simulink subsystem "Controls"  (R2024b)
settings: Solver=VariableStepAuto  StartTime=0.0  StopTime=10.0  RelTol=1e-3
undefined symbols (not defined in the file): D1, DiscIntNeverNeededParam, lag, Tctrl, test_alpha, Ts, Yg
libraries: powerlib_extras x74, simulink x10
(part 5 of 7)

== system Controls/fault_trigger/faultgen/faultgen ==
  t : Inport
  Tstat : Inport  Port=2
  Tdur : Inport  Port=3
  Add : Sum
  Logical Operator : Logic  AllPortsSameDT=off  OutDataTypeStr=boolean
  Relational Operator1 : RelationalOperator  Operator=<=  OutDataTypeStr=boolean  InputSameDT=off
  Relational Operatr : RelationalOperator  OutDataTypeStr=boolean  InputSameDT=off
  fault : Outport
  wires:
  Tstat/1 -> Add/1, Relational Operatr/2
  Tdur/1 -> Add/2
  Logical Operator/1 -> fault/1
  t/1 -> Relational Operator1/1, Relational Operatr/1
  Relational Operatr/1 -> Logical Operator/1
  Relational Operator1/1 -> Logical Operator/2
  Add/1 -> Relational Operator1/2

== system Controls/fault_trigger/faultgen/sawtooth ==
  Taqu : Inport
  pules : Inport  Port=2
  Constant : Constant
  Data Type Conversion : DataTypeConversion  SaturateOnIntegerOverflow=off  RndMeth=Floor
  Discrete-Time Integrator : DiscreteIntegrator  ExternalReset=rising  SampleTime=-1  ICPrevOutput=DiscIntNeverNeededParam  ICPrevScaledInput=DiscIntNeverNeededParam
  Logical Operator : Logic  AllPortsSameDT=off
  Relational Operator : RelationalOperator  OutDataTypeStr=boolean  InputSameDT=off
  Unit Delay : UnitDelay  SampleTime=Ts  HasFrameUpgradeWarning=on
  sawtooth : Outport
  trig : Outport  Port=2
  wires:
  Unit Delay/1 -> Relational Operator/1
  Data Type Conversion/1 -> trig/1
  Taqu/1 -> Relational Operator/2
  pules/1 -> Logical Operator/1
  Relational Operator/1 -> Logical Operator/2
  Logical Operator/1 -> Data Type Conversion/1, Discrete-Time Integrator/2
  Discrete-Time Integrator/1 -> sawtooth/1, Unit Delay/1
  Constant/1 -> Discrete-Time Integrator/1

== system Controls/Pole 1 Inverter Control and Protection/Inverter Current //Voltage//Gamma Controller /Current Regulator/Kp Linearisation ==
  note: Kp Linearization
  Alpha_lin : Inport
  Kp : Inport  Port=2
  Inv : Inport  Port=3
  Min_lin : Inport  Port=4
  Max_lin : Inport  Port=5
  Constant3 : Constant  Value=On_lin
  Data Type Conversion : DataTypeConversion  OutDataTypeStr=boolean
  Logical Operator : Logic  Operator=NOT
  Logical Operator1 : Logic  Operator=NOT
  Math Function : Math  Operator=reciprocal  SignedPower=on
  Prod2 : Product  Inputs=3  InputSameDT=on  SaturateOnIntegerOverflow=on  OutDataTypeStr=Inherit: Same as first input
  S6 : Subsystem  mask(Limiter with External Limits){}
      mask Display: disp('      Limiter\n')
  Switch : Switch  Threshold=0.5
  Switch1 : Switch  Threshold=0.5
  Trigonometric Function : Trigonometry
  Trigonometric Function1 : Trigonometry
  k : Gain  Gain=pi/180  SaturateOnIntegerOverflow=on  OutDataTypeStr=Inherit: Same as input  ParamDataTypeStr=Inherit: Same as input
  k1 : Gain  Gain=pi/180  SaturateOnIntegerOverflow=on  OutDataTypeStr=Inherit: Same as input  ParamDataTypeStr=Inherit: Same as input
  Kp_lin : Outport  InitialOutput=0
  wires:
  Data Type Conversion/1 -> Logical Operator1/1
  Constant3/1 -> Data Type Conversion/1
  Min_lin/1 -> S6/3(MIN), Switch/1
  Max_lin/1 -> S6/1(MAX), Switch/3
  Alpha_lin/1 -> S6/2(In)
  Math Function/1 -> Prod2/2
  Trigonometric Function1/1 -> Math Function/1
  k/1 -> Trigonometric Function1/1
  Kp/1 -> Prod2/3, Switch1/1
  Inv/1 -> Logical Operator/1
  Logical Operator/1 -> Switch/2
  Trigonometric Function/1 -> Prod2/1
  S6/1("  ") -> k/1
  k1/1 -> Trigonometric Function/1
  Switch/1 -> k1/1
  Switch1/1 -> Kp_lin/1
  Prod2/1 -> Switch1/3
  Logical Operator1/1 -> Switch1/2  "Off"

== system Controls/Pole 1 Inverter Control and Protection/Inverter Current //Voltage//Gamma Controller /Current Regulator/S16 ==
  note: INTEGRATOR with External limits & Reset & Hold
  note: Gain * dt
  Max : Inport
  Min : Inport  Port=2
  In : Inport  Port=3
  Reset : Inport  Port=4
  Hold : Inport  Port=5
  Reset Value : Inport  Port=6
  Gain1 : Gain  Gain=k*dt  SaturateOnIntegerOverflow=on  OutDataTypeStr=Inherit: Same as input  ParamDataTypeStr=Inherit: Same as input
  IC = ic : UnitDelay  InitialCondition=ic  SampleTime=dt  HasFrameUpgradeWarning=on
  Logical Operator4 : Logic  Operator=OR
  MinMax : MinMax  Inputs=2  InputSameDT=on  SaturateOnIntegerOverflow=on
  MinMax1 : MinMax  Function=max  Inputs=2  InputSameDT=on  SaturateOnIntegerOverflow=on
  S6 : Subsystem  mask(Limiter with External Limits){}
      mask Display: disp('      Limiter\n')
  Sum : Sum  InputSameDT=on  SaturateOnIntegerOverflow=on  OutDataTypeStr=Inherit: Same as first input
  Switch2 : Switch  Threshold=0.5
  Switch3 : Switch  Threshold=0.5
  Switch7 : Switch  Threshold=0.5
  Out : Outport  InitialOutput=0
  wires:
  Gain1/1 -> Sum/1
  In/1 -> Gain1/1
  Sum/1 -> S6/2(In)
  S6/1("  ") -> Out/1, IC = ic/1
  Hold/1 -> Logical Operator4/1
  Reset/1 -> Switch7/2, Logical Operator4/2
  Logical Operator4/1 -> Switch2/2, Switch3/2
  Switch2/1 -> MinMax/1
  Max/1 -> Switch2/3, MinMax/2
  Reset Value/1 -> Switch7/1
  MinMax/1 -> S6/1(MAX)
  MinMax1/1 -> S6/3(MIN)
  Switch3/1 -> MinMax1/1
  Min/1 -> Switch3/3, MinMax1/2
  IC = ic/1 -> Switch7/3
  Switch7/1 -> Switch2/1, Sum/2, Switch3/1

== system Controls/Pole 1 Inverter Control and Protection/Inverter Current //Voltage//Gamma Controller /Current Regulator/S6 ==
  note: Limiter
      | with external
      | limits
  MAX : Inport
  In : Inport  Port=2
  MIN : Inport  Port=3
  MinMax : MinMax  Function=max  Inputs=2  InputSameDT=on  SaturateOnIntegerOverflow=on
  MinMax1 : MinMax  Inputs=2  InputSameDT=on  SaturateOnIntegerOverflow=on
  "  " : Outport  InitialOutput=0
  wires:
  In/1 -> MinMax1/2
  MinMax/1 -> "  "/1
  MIN/1 -> MinMax/1
  MAX/1 -> MinMax1/1
  MinMax1/1 -> MinMax/2

== system Controls/Pole 1 Inverter Control and Protection/Inverter Current //Voltage//Gamma Controller /Gamma Error/S6 ==
  note: Limiter
      | with external
      | limits
  MAX : Inport
  In : Inport  Port=2
  MIN : Inport  Port=3
  MinMax : MinMax  Function=max  Inputs=2  InputSameDT=on  SaturateOnIntegerOverflow=on
  MinMax1 : MinMax  Inputs=2  InputSameDT=on  SaturateOnIntegerOverflow=on
  "  " : Outport  InitialOutput=0
  wires:
  MinMax1/1 -> MinMax/2
  MAX/1 -> MinMax1/1
  MIN/1 -> MinMax/1
  MinMax/1 -> "  "/1
  In/1 -> MinMax1/2

== system Controls/Pole 1 Inverter Control and Protection/Inverter Current //Voltage//Gamma Controller /Gamma Regulator/Gamma Regulator ==
  note: PI Regulator With external limits (Linearized Kp) (Discrete)
  Max_i : Inport
  Min_i : Inport  Port=2
  ERR : Inport  Port=3
  Max_pi : Inport  Port=4
  Min_pi : Inport  Port=5
  Alpha_lin : Inport  Port=6
  Max_lin : Inport  Port=7
  Min_lin : Inport  Port=8
  Inv : Inport  Port=9
  Kp : Inport  Port=10
  Ki : Inport  Port=11
  Ground : Ground
  KI (deg per pu per s) : Gain  Gain=Ki  SaturateOnIntegerOverflow=on  OutDataTypeStr=Inherit: Same as input  ParamDataTypeStr=Inherit: Same as input
  Kp (deg per pu) : Constant  Value=Kp
  Kp Linearisation : Subsystem
  Prod : Product  InputSameDT=on  SaturateOnIntegerOverflow=on  OutDataTypeStr=Inherit: Same as first input
  Prod1 : Product  InputSameDT=on  SaturateOnIntegerOverflow=on  OutDataTypeStr=Inherit: Same as first input
  S16 : Subsystem  mask(Integrator  With  External  Dynamic  Limits (Discrete)){k=1, ic=IC_i, st=pas}
      mask prompts: k "Gain:"; ic "Initial Condition:"; st "Sample time: (s)"
      mask Display: disp('Integrator\nwith\nExternal Limits\nGain & Reset & Hold\n(Discrete)')
  S6 : Subsystem  mask(Limiter with External Limits){}
      mask Display: disp('      Limiter\n')
  Sum : Sum  InputSameDT=on  SaturateOnIntegerOverflow=on  OutDataTypeStr=Inherit: Same as first input
  Alpha_ord : Outport  InitialOutput=0
  wires:
  Prod1/1 -> S16/3(In)
  Ki/1 -> Prod1/2
  Kp/1 -> Kp Linearisation/2(Kp)
  Alpha_lin/1 -> Kp Linearisation/1(Alpha_lin)
  S6/1("  ") -> Alpha_ord/1
  Kp Linearisation/1(Kp_lin) -> Prod/1
  Max_i/1 -> S16/1(Max)
  Min_i/1 -> S16/2(Min)
  Sum/1 -> S6/2(In)
  Max_pi/1 -> S6/1(MAX)
  Min_pi/1 -> S6/3(MIN)
  S16/1(Out) -> Sum/2
  ERR/1 -> Prod1/1, KI (deg per pu per s)/1, Prod/2
  Ground/1 -> S16/4(Reset), S16/5(Hold), S16/6(Reset Value)
  Inv/1 -> Kp Linearisation/3(Inv)
  Max_lin/1 -> Kp Linearisation/5(Max_lin)
  Min_lin/1 -> Kp Linearisation/4(Min_lin)
  Prod/1 -> Sum/1

== system Controls/Pole 1 Inverter Control and Protection/Inverter Current //Voltage//Gamma Controller /Voltage Dependant Current Order Limiter/PB_R ==
  note: Silvano Casoria
      | Laboratoire simulation de reseaux, IREQ
  note: LOW PASS Filter & RESET
      | (Zoh methode)
  "In " : Inport
  Reset : Inport  Port=2
  T : Inport  Port=3
  Constant : Constant  Value=dt
  IC= ic : UnitDelay  InitialCondition=ic  SampleTime=dt  HasFrameUpgradeWarning=on
  Math Function : Math  Operator=reciprocal  SignedPower=on
  Product : Product  Inputs=3  InputSameDT=on  SaturateOnIntegerOverflow=on  OutDataTypeStr=Inherit: Same as first input
  Sum : Sum  Inputs=+-  InputSameDT=on  SaturateOnIntegerOverflow=on  OutDataTypeStr=Inherit: Same as first input
  Sum1 : Sum  InputSameDT=on  SaturateOnIntegerOverflow=on
  Switch : Switch  Threshold=0.5
  Out : Outport  InitialOutput=0
  wires:
  IC= ic/1 -> Sum/2, Sum1/2
  "In "/1 -> Sum/1, Switch/1
  Reset/1 -> Switch/2
  Sum1/1 -> Out/1, Switch/3
  Switch/1 -> IC= ic/1
  Product/1 -> Sum1/1
  Sum/1 -> Product/2
  Math Function/1 -> Product/1
  T/1 -> Math Function/1
  Constant/1 -> Product/3

== system Controls/Pole 1 Inverter Control and Protection/Inverter Current //Voltage//Gamma Controller /Voltage Error/S6 ==
  note: Limiter
      | with external
      | limits
  MAX : Inport
  In : Inport  Port=2
  MIN : Inport  Port=3
  MinMax : MinMax  Function=max  Inputs=2  InputSameDT=on  SaturateOnIntegerOverflow=on
  MinMax1 : MinMax  Inputs=2  InputSameDT=on  SaturateOnIntegerOverflow=on
  "  " : Outport  InitialOutput=0
  wires:
  In/1 -> MinMax1/2
  MinMax/1 -> "  "/1
  MIN/1 -> MinMax/1
  MAX/1 -> MinMax1/1
  MinMax1/1 -> MinMax/2

== system Controls/Pole 1 Inverter Control and Protection/Inverter Current //Voltage//Gamma Controller /Voltage Regulator/Voltage Regulator ==
  note: PI Regulator With external limits (Linearized Kp) (Discrete)
  Max_i : Inport
  Min_i : Inport  Port=2
  ERR : Inport  Port=3
  Max_pi : Inport  Port=4
  Min_pi : Inport  Port=5
  Alpha_lin : Inport  Port=6
  Max_lin : Inport  Port=7
  Min_lin : Inport  Port=8
  Inv : Inport  Port=9
  Kp : Inport  Port=10
  Ki : Inport  Port=11
  Ground : Ground
  KI (deg per pu per s) : Gain  Gain=Ki  SaturateOnIntegerOverflow=on  OutDataTypeStr=Inherit: Same as input  ParamDataTypeStr=Inherit: Same as input
  Kp (deg per pu) : Constant  Value=Kp
  Kp Linearisation : Subsystem
  Prod : Product  InputSameDT=on  SaturateOnIntegerOverflow=on  OutDataTypeStr=Inherit: Same as first input
  Prod1 : Product  InputSameDT=on  SaturateOnIntegerOverflow=on  OutDataTypeStr=Inherit: Same as first input
  S16 : Subsystem  mask(Integrator  With  External  Dynamic  Limits (Discrete)){k=1, ic=IC_i, st=pas}
      mask prompts: k "Gain:"; ic "Initial Condition:"; st "Sample time: (s)"
      mask Display: disp('Integrator\nwith\nExternal Limits\nGain & Reset & Hold\n(Discrete)')
  S6 : Subsystem  mask(Limiter with External Limits){}
      mask Display: disp('      Limiter\n')
  Sum : Sum  InputSameDT=on  SaturateOnIntegerOverflow=on  OutDataTypeStr=Inherit: Same as first input
  Alpha_ord : Outport  InitialOutput=0
  wires:
  Prod1/1 -> S16/3(In)
  Ki/1 -> Prod1/2
  Kp/1 -> Kp Linearisation/2(Kp)
  Prod/1 -> Sum/1
  Min_lin/1 -> Kp Linearisation/4(Min_lin)
  Max_lin/1 -> Kp Linearisation/5(Max_lin)
  Inv/1 -> Kp Linearisation/3(Inv)
  Ground/1 -> S16/6(Reset Value), S16/5(Hold), S16/4(Reset)
  ERR/1 -> Prod1/1, Prod/2, KI (deg per pu per s)/1
  S16/1(Out) -> Sum/2
  Min_pi/1 -> S6/3(MIN)
  Max_pi/1 -> S6/1(MAX)
  Sum/1 -> S6/2(In)
  Min_i/1 -> S16/2(Min)
  Max_i/1 -> S16/1(Max)
  Kp Linearisation/1(Kp_lin) -> Prod/1
  S6/1("  ") -> Alpha_ord/1
  Alpha_lin/1 -> Kp Linearisation/1(Alpha_lin)

== system Controls/Pole 1 Inverter Control and Protection/Inverter Protections/Commutation Failure Prevention Control (CFPREV)/Enabled Subsystem ==
  note: Fast initialisation
      | for simulation
  note: Commutation failure Prevention Control (CFPREV)
  note: Silvano Casoria
      | Power System Laboratory, IREQ
      | Hydro-Quebec
  note: Ref. "A Novel Method to Mitigate Commutation Failures in HVDC Systems,"
      | Lidong Zhang, Lars Dofnas ABB Utilities Power System Technology,
      | Proceedings PowerCon 2002, Volume: 1 , 13-17 Oct. 2002,  Page(s): 51-56 vol.1
  Uabc (pu) : Inport
  Enable : EnablePort
  AB_LEVEL : Constant  Value=ab_level
  ALPFA_BETA_SUM : Fcn  Expr=sqrt(u[1]^2+u[2]^2)
  ALPFA_BETA_SUM1 : Fcn  Expr=abs(u[3]) * 3
  C : Constant  Value=filt_tc
  C1 : Constant  Value=1/(fn)
  CLARK : Subsystem
  Gain : Gain  Gain=ab_gain  SaturateOnIntegerOverflow=on  OutDataTypeStr=Inherit: Same as input  ParamDataTypeStr=Inherit: Same as input
  "Gain  " : Gain  Gain=z_gain  SaturateOnIntegerOverflow=on  OutDataTypeStr=Inherit: Same as input  ParamDataTypeStr=Inherit: Same as input
  Ground : Ground
  LP T= 0.03 : powerlib_extras/Discrete  Control Blocks/Discrete 1st-Order Filter  FilterType=Lowpass  Tc=0.03  Ts=Ts  Initialize=off  Vac_Init=[0.8 -25 60]*0  Vdc_Init=filt_ic  PlotResponse=off  param1=[1 500 0.1]
  Max: 1 pu Min = 0 : Saturate  UpperLimit=1.0  LowerLimit=0
  MinMax2 : MinMax  Function=max  InputSameDT=on  SaturateOnIntegerOverflow=on
  MinMax3 : MinMax  Function=max  Inputs=2  InputSameDT=on  SaturateOnIntegerOverflow=on
  MinMax4 : MinMax  Function=max  Inputs=2  InputSameDT=on  SaturateOnIntegerOverflow=on
  MinMax5 : MinMax  Function=max  InputSameDT=on  SaturateOnIntegerOverflow=on
  PB_R : Subsystem  mask(Low Pass Filter With Reset (discrete: Zoh method, Forward Euler)){ic=1, dt=Ts}
      mask prompts: ic "Initial condition:"; dt "Sample time (s)"
      mask help:
      | The output will be reset to the input value (Time constant = 0)  during the input (2) is True. The Time constant (T) is defined by
      | input (3).
      mask Display:
      | plot(0,0,100,100,[90,80,70,60,50,40,29,20,10],[60,55,52,55,60,65,67,65,60],[89,80,71,60,50,40,30,20,10],[40,35,32,35,40,45,47,45,40],[56,44],[70,50]);
      | disp('\n\nD')
  Relational Operator : RelationalOperator  Operator=>  InputSameDT=off
  Relational Operator1 : RelationalOperator  Operator=>  InputSameDT=off
  Sum : Sum  Inputs=+-  SaturateOnIntegerOverflow=on
  Switch : Switch  Threshold=0.5  InputSameDT=off
  Switch1 : Switch  Threshold=0.5  InputSameDT=off
  Switch2 : Switch  Threshold=0.5  InputSameDT=off
  T_ss : Step  Time=T_ss  Before=1  After=0  SampleTime=Ts
  Tapped Delay : simulink/Discrete/Tapped Delay  vinit=0.0  samptime=Ts  NumDelays=fix(T_periode/Ts)  DelayOrder=Newest  includeCurrent=off
  Tapped Delay1 : simulink/Discrete/Tapped Delay  vinit=0.0  samptime=Ts  NumDelays=fix(T_periode/Ts)  DelayOrder=Newest  includeCurrent=off
  ZERO : Constant  Value=0
  ZERO1 : Constant  Value=0
  Z_LEVEL : Constant  Value=z_level
  AMIN_CFPREV (deg) : Outport
  wires:
  Tapped Delay/1 -> MinMax5/1
  Ground/1 -> PB_R/2(Reset)
  C1/1 -> Switch2/1
  T_ss/1 -> Switch2/2
  C/1 -> Switch2/3
  Switch2/1 -> PB_R/3(T)
  PB_R/1(Out) -> Sum/1
  Uabc (pu)/1 -> CLARK/1(abc)
  CLARK/1(ab0) -> ALPFA_BETA_SUM1/1, ALPFA_BETA_SUM/1
  Switch1/1 -> MinMax3/2  "Z MIN"
  Switch/1 -> MinMax3/1  "AB MIN"
  ZERO1/1 -> Switch1/3
  "Gain  "/1 -> Switch1/1  "Z_AMIN"
  Relational Operator1/1 -> Switch1/2  "Z_DET"
  Max: 1 pu Min = 0/1 -> "Gain  "/1
  MinMax2/1 -> Max: 1 pu Min = 0/1
  Tapped Delay1/1 -> MinMax2/1
  Z_LEVEL/1 -> Relational Operator1/2
  ALPFA_BETA_SUM1/1 -> Tapped Delay1/1, Relational Operator1/1  "Z_DIFF"
  ZERO/1 -> Switch/3
  Gain/1 -> Switch/1  "AB_AMIN"
  MinMax5/1 -> Gain/1
  Relational Operator/1 -> Switch/2  "AB_DET"
  AB_LEVEL/1 -> Relational Operator/2
  Sum/1 -> Tapped Delay/1, Relational Operator/1
  ALPFA_BETA_SUM/1 -> PB_R/1("In "), Sum/2
  MinMax3/1 -> MinMax4/2, LP T= 0.03/1
  LP T= 0.03/1 -> MinMax4/1
  MinMax4/1 -> AMIN_CFPREV (deg)/1

== system Controls/Pole 1 Inverter Control and Protection/Inverter Protections/Low AC Voltage Detection (LACVD)/Enabled Subsystem ==
  note: Low AC Voltage Detection
  note: Silvano Casoria
      | Power System Laboratory, IREQ
      | Hydro-Quebec
  Uac (pu) : Inport
  "Off Delay " : powerlib_extras/Discrete  Control Blocks/Discrete On//Off Delay  type_delay=Off delay  delay=0.009  ic=0  Ts=dt
  On Delay : powerlib_extras/Discrete  Control Blocks/Discrete On//Off Delay  type_delay=On delay  delay=0.014  ic=0  Ts=dt
  "On Delay " : powerlib_extras/Discrete  Control Blocks/Discrete On//Off Delay  type_delay=On delay  delay=0.001  ic=0  Ts=dt
  REF 1 (pu) : Constant  Value=Ref_1
  Relational Operator1 : RelationalOperator  Operator=<=
  Low_AC_Voltage : Outport
  wires:
  Uac (pu)/1 -> Relational Operator1/1
  On Delay/1 -> Low_AC_Voltage/1
  REF 1 (pu)/1 -> Relational Operator1/2
  "Off Delay "/1 -> On Delay/1
  "On Delay "/1 -> "Off Delay "/1
  Relational Operator1/1 -> "On Delay "/1

== system Controls/Pole 1 Rectifier Control and Protection/Rectifier Controller/Current Regulator/Kp Linearisation ==
  note: Kp Linearization
  Alpha_lin : Inport
  Kp : Inport  Port=2
  Inv : Inport  Port=3
  Min_lin : Inport  Port=4
  Max_lin : Inport  Port=5
  Constant3 : Constant  Value=On_lin
  Data Type Conversion : DataTypeConversion  OutDataTypeStr=boolean
  Logical Operator : Logic  Operator=NOT
  Logical Operator1 : Logic  Operator=NOT
  Math Function : Math  Operator=reciprocal  SignedPower=on
  Prod2 : Product  Inputs=3  InputSameDT=on  SaturateOnIntegerOverflow=on  OutDataTypeStr=Inherit: Same as first input
  S6 : Subsystem  mask(Limiter with External Limits){}
      mask Display: disp('      Limiter\n')
  Switch : Switch  Threshold=0.5
  Switch1 : Switch  Threshold=0.5
  Trigonometric Function : Trigonometry
  Trigonometric Function1 : Trigonometry
  k : Gain  Gain=pi/180  SaturateOnIntegerOverflow=on  OutDataTypeStr=Inherit: Same as input  ParamDataTypeStr=Inherit: Same as input
  k1 : Gain  Gain=pi/180  SaturateOnIntegerOverflow=on  OutDataTypeStr=Inherit: Same as input  ParamDataTypeStr=Inherit: Same as input
  Kp_lin : Outport  InitialOutput=0
  wires:
  Data Type Conversion/1 -> Logical Operator1/1
  Constant3/1 -> Data Type Conversion/1
  Min_lin/1 -> S6/3(MIN), Switch/1
  Max_lin/1 -> S6/1(MAX), Switch/3
  Alpha_lin/1 -> S6/2(In)
  Math Function/1 -> Prod2/2
  Trigonometric Function1/1 -> Math Function/1
  k/1 -> Trigonometric Function1/1
  Kp/1 -> Prod2/3, Switch1/1
  Inv/1 -> Logical Operator/1
  Logical Operator/1 -> Switch/2
  Trigonometric Function/1 -> Prod2/1
  S6/1("  ") -> k/1
  k1/1 -> Trigonometric Function/1
  Switch/1 -> k1/1
  Switch1/1 -> Kp_lin/1
  Prod2/1 -> Switch1/3
  Logical Operator1/1 -> Switch1/2  "Off"

== system Controls/Pole 1 Rectifier Control and Protection/Rectifier Controller/Current Regulator/S16 ==
  note: INTEGRATOR with External limits & Reset & Hold
  note: Gain * dt
  Max : Inport
  Min : Inport  Port=2
  In : Inport  Port=3
  Reset : Inport  Port=4
  Hold : Inport  Port=5
  Reset Value : Inport  Port=6
  Gain1 : Gain  Gain=k*dt  SaturateOnIntegerOverflow=on  OutDataTypeStr=Inherit: Same as input  ParamDataTypeStr=Inherit: Same as input
  IC = ic : UnitDelay  InitialCondition=ic  SampleTime=dt  HasFrameUpgradeWarning=on
  Logical Operator4 : Logic  Operator=OR
  MinMax : MinMax  Inputs=2  InputSameDT=on  SaturateOnIntegerOverflow=on
  MinMax1 : MinMax  Function=max  Inputs=2  InputSameDT=on  SaturateOnIntegerOverflow=on
  S6 : Subsystem  mask(Limiter with External Limits){}
      mask Display: disp('      Limiter\n')
  Sum : Sum  InputSameDT=on  SaturateOnIntegerOverflow=on  OutDataTypeStr=Inherit: Same as first input
  Switch2 : Switch  Threshold=0.5
  Switch3 : Switch  Threshold=0.5
  Switch7 : Switch  Threshold=0.5
  Out : Outport  InitialOutput=0
  wires:
  Gain1/1 -> Sum/1
  In/1 -> Gain1/1
  Sum/1 -> S6/2(In)
  S6/1("  ") -> Out/1, IC = ic/1
  Hold/1 -> Logical Operator4/1
  Reset/1 -> Switch7/2, Logical Operator4/2
  Logical Operator4/1 -> Switch2/2, Switch3/2
  Switch2/1 -> MinMax/1
  Max/1 -> Switch2/3, MinMax/2
  Reset Value/1 -> Switch7/1
  MinMax/1 -> S6/1(MAX)
  MinMax1/1 -> S6/3(MIN)
  Switch3/1 -> MinMax1/1
  Min/1 -> Switch3/3, MinMax1/2
  IC = ic/1 -> Switch7/3
  Switch7/1 -> Switch2/1, Sum/2, Switch3/1

== system Controls/Pole 1 Rectifier Control and Protection/Rectifier Controller/Current Regulator/S6 ==
  note: Limiter
      | with external
      | limits
  MAX : Inport
  In : Inport  Port=2
  MIN : Inport  Port=3
  MinMax : MinMax  Function=max  Inputs=2  InputSameDT=on  SaturateOnIntegerOverflow=on
  MinMax1 : MinMax  Inputs=2  InputSameDT=on  SaturateOnIntegerOverflow=on
  "  " : Outport  InitialOutput=0
  wires:
  In/1 -> MinMax1/2
  MinMax/1 -> "  "/1
  MIN/1 -> MinMax/1
  MAX/1 -> MinMax1/1
  MinMax1/1 -> MinMax/2

== system Controls/Pole 1 Rectifier Control and Protection/Rectifier Controller/Gamma Error/S6 ==
  note: Limiter
      | with external
      | limits
  MAX : Inport
  In : Inport  Port=2
  MIN : Inport  Port=3
  MinMax : MinMax  Function=max  Inputs=2  InputSameDT=on  SaturateOnIntegerOverflow=on
  MinMax1 : MinMax  Inputs=2  InputSameDT=on  SaturateOnIntegerOverflow=on
  "  " : Outport  InitialOutput=0
  wires:
  MinMax1/1 -> MinMax/2
  MAX/1 -> MinMax1/1
  MIN/1 -> MinMax/1
  MinMax/1 -> "  "/1
  In/1 -> MinMax1/2

== system Controls/Pole 1 Rectifier Control and Protection/Rectifier Controller/Gamma Regulator/Gamma Regulator ==
  note: PI Regulator With external limits (Linearized Kp) (Discrete)
  Max_i : Inport
  Min_i : Inport  Port=2
  ERR : Inport  Port=3
  Max_pi : Inport  Port=4
  Min_pi : Inport  Port=5
  Alpha_lin : Inport  Port=6
  Max_lin : Inport  Port=7
  Min_lin : Inport  Port=8
  Inv : Inport  Port=9
  Kp : Inport  Port=10
  Ki : Inport  Port=11
  Ground : Ground
  KI (deg per pu per s) : Gain  Gain=Ki  SaturateOnIntegerOverflow=on  OutDataTypeStr=Inherit: Same as input  ParamDataTypeStr=Inherit: Same as input
  Kp (deg per pu) : Constant  Value=Kp
  Kp Linearisation : Subsystem
  Prod : Product  InputSameDT=on  SaturateOnIntegerOverflow=on  OutDataTypeStr=Inherit: Same as first input
  Prod1 : Product  InputSameDT=on  SaturateOnIntegerOverflow=on  OutDataTypeStr=Inherit: Same as first input
  S16 : Subsystem  mask(Integrator  With  External  Dynamic  Limits (Discrete)){k=1, ic=IC_i, st=pas}
      mask prompts: k "Gain:"; ic "Initial Condition:"; st "Sample time: (s)"
      mask Display: disp('Integrator\nwith\nExternal Limits\nGain & Reset & Hold\n(Discrete)')
  S6 : Subsystem  mask(Limiter with External Limits){}
      mask Display: disp('      Limiter\n')
  Sum : Sum  InputSameDT=on  SaturateOnIntegerOverflow=on  OutDataTypeStr=Inherit: Same as first input
  Alpha_ord : Outport  InitialOutput=0
  wires:
  Prod1/1 -> S16/3(In)
  Ki/1 -> Prod1/2
  Kp/1 -> Kp Linearisation/2(Kp)
  Alpha_lin/1 -> Kp Linearisation/1(Alpha_lin)
  S6/1("  ") -> Alpha_ord/1
  Kp Linearisation/1(Kp_lin) -> Prod/1
  Max_i/1 -> S16/1(Max)
  Min_i/1 -> S16/2(Min)
  Sum/1 -> S6/2(In)
  Max_pi/1 -> S6/1(MAX)
  Min_pi/1 -> S6/3(MIN)
  S16/1(Out) -> Sum/2
  ERR/1 -> Prod1/1, KI (deg per pu per s)/1, Prod/2
  Ground/1 -> S16/4(Reset), S16/5(Hold), S16/6(Reset Value)
  Inv/1 -> Kp Linearisation/3(Inv)
  Max_lin/1 -> Kp Linearisation/5(Max_lin)
  Min_lin/1 -> Kp Linearisation/4(Min_lin)
  Prod/1 -> Sum/1

== system Controls/Pole 1 Rectifier Control and Protection/Rectifier Controller/Voltage Dependant Current Order Limiter/PB_R ==
  note: Silvano Casoria
      | Laboratoire simulation de reseaux, IREQ
  note: LOW PASS Filter & RESET
      | (Zoh methode)
  "In " : Inport
  Reset : Inport  Port=2
  T : Inport  Port=3
  Constant : Constant  Value=dt
  IC= ic : UnitDelay  InitialCondition=ic  SampleTime=dt  HasFrameUpgradeWarning=on
  Math Function : Math  Operator=reciprocal  SignedPower=on
  Product : Product  Inputs=3  InputSameDT=on  SaturateOnIntegerOverflow=on  OutDataTypeStr=Inherit: Same as first input
  Sum : Sum  Inputs=+-  InputSameDT=on  SaturateOnIntegerOverflow=on  OutDataTypeStr=Inherit: Same as first input
  Sum1 : Sum  InputSameDT=on  SaturateOnIntegerOverflow=on
  Switch : Switch  Threshold=0.5
  Out : Outport  InitialOutput=0
  wires:
  IC= ic/1 -> Sum/2, Sum1/2
  "In "/1 -> Sum/1, Switch/1
  Reset/1 -> Switch/2
  Sum1/1 -> Out/1, Switch/3
  Switch/1 -> IC= ic/1
  Product/1 -> Sum1/1
  Sum/1 -> Product/2
  Math Function/1 -> Product/1
  T/1 -> Math Function/1
  Constant/1 -> Product/3

== system Controls/Pole 1 Rectifier Control and Protection/Rectifier Controller/Voltage Error/S6 ==
  note: Limiter
      | with external
      | limits
  MAX : Inport
  In : Inport  Port=2
  MIN : Inport  Port=3
  MinMax : MinMax  Function=max  Inputs=2  InputSameDT=on  SaturateOnIntegerOverflow=on
  MinMax1 : MinMax  Inputs=2  InputSameDT=on  SaturateOnIntegerOverflow=on
  "  " : Outport  InitialOutput=0
  wires:
  In/1 -> MinMax1/2
  MinMax/1 -> "  "/1
  MIN/1 -> MinMax/1
  MAX/1 -> MinMax1/1
  MinMax1/1 -> MinMax/2

== system Controls/Pole 1 Rectifier Control and Protection/Rectifier Controller/Voltage Regulator/Voltage Regulator ==
  note: PI Regulator With external limits (Linearized Kp) (Discrete)
  Max_i : Inport
  Min_i : Inport  Port=2
  ERR : Inport  Port=3
  Max_pi : Inport  Port=4
  Min_pi : Inport  Port=5
  Alpha_lin : Inport  Port=6
  Max_lin : Inport  Port=7
  Min_lin : Inport  Port=8
  Inv : Inport  Port=9
  Kp : Inport  Port=10
  Ki : Inport  Port=11
  Ground : Ground
  KI (deg per pu per s) : Gain  Gain=Ki  SaturateOnIntegerOverflow=on  OutDataTypeStr=Inherit: Same as input  ParamDataTypeStr=Inherit: Same as input
  Kp Linearisation : Subsystem
  Prod : Product  InputSameDT=on  SaturateOnIntegerOverflow=on  OutDataTypeStr=Inherit: Same as first input
  Prod1 : Product  InputSameDT=on  SaturateOnIntegerOverflow=on  OutDataTypeStr=Inherit: Same as first input
  S16 : Subsystem  mask(Integrator  With  External  Dynamic  Limits (Discrete)){k=1, ic=IC_i, st=pas}
      mask prompts: k "Gain:"; ic "Initial Condition:"; st "Sample time: (s)"
      mask Display: disp('Integrator\nwith\nExternal Limits\nGain & Reset & Hold\n(Discrete)')
  S6 : Subsystem  mask(Limiter with External Limits){}
      mask Display: disp('      Limiter\n')
  Sum : Sum  InputSameDT=on  SaturateOnIntegerOverflow=on  OutDataTypeStr=Inherit: Same as first input
  Alpha_ord : Outport  InitialOutput=0
  wires:
  Prod1/1 -> S16/3(In)
  Ki/1 -> Prod1/2
  Kp/1 -> Kp Linearisation/2(Kp)
  Prod/1 -> Sum/1
  Min_lin/1 -> Kp Linearisation/4(Min_lin)
  Max_lin/1 -> Kp Linearisation/5(Max_lin)
  Inv/1 -> Kp Linearisation/3(Inv)
  Ground/1 -> S16/6(Reset Value), S16/5(Hold), S16/4(Reset)
  ERR/1 -> Prod1/1, Prod/2, KI (deg per pu per s)/1
  S16/1(Out) -> Sum/2
  Min_pi/1 -> S6/3(MIN)
  Max_pi/1 -> S6/1(MAX)
  Sum/1 -> S6/2(In)
  Min_i/1 -> S16/2(Min)
  Max_i/1 -> S16/1(Max)
  Kp Linearisation/1(Kp_lin) -> Prod/1
  S6/1("  ") -> Alpha_ord/1
  Alpha_lin/1 -> Kp Linearisation/1(Alpha_lin)

== system Controls/Pole 1 Rectifier Control and Protection/Rectifier Protections/DC Fault Protection (DCPROT)/Enabled Subsystem ==
  note: DC Fault Protection (only in Rectifier)
  note: Silvano Casoria
      | Power System Laboratory, IREQ
      | Hydro-Quebec
  VdL (pu) : Inport
  Deblocked : Inport  Port=2  OutDataTypeStr=boolean
  Lock : Inport  Port=3
  Data Type Conversion : DataTypeConversion  OutDataTypeStr=boolean
  Discrete Off Delay : Subsystem  AncestorBlock=|  mask(Discrete On/Off Delay){type_delay=Off delay, delay=0.160, ic=0, Ts=dt}
      | powerlib_extras/Discrete 
      | Control Blocks/Discrete
      | On//Off Delay
      mask prompts: type_delay "Type:"; delay "Time delay:"; ic "Input at t = -Ts (0/1):"; Ts "Sample time Ts:"
      mask help:
      | Apply a delay on the input signal when the input changes to TRUE (1) or FALSE (0).
      |
      | On delay: When the input becomes TRUE, the output becomes TRUE after the specified time delay as long as the input is still TRUE. If the input becomes FALSE before the time delay has expired , the output stays FALSE.
      |
      | Off delay: When the input becomes FALSE, the output becomes FALSE after the specified time delay as long as the input is still FALSE. If the input becomes TRUE before the time delay has expired , the output stays TRUE.
      |
      | The input value (0/1) at time step preceding t=0 is specified by the parameter "input at t = -Ts".
      mask init:
      | str=sprintf('%g %c',delay,'s');
      | power_initmask();
      mask Help: This block is part of a subset of blocks in the Extras library that does not have documentation associated with it, other than the block mask description.
      mask TypeOptions type_delay: On delay | Off delay
      mask Display:
      | plot(0,0,100,100,[10,10,10,90,90,90],[60,40,50,50,40,60]);
      | text(25+(type_delay-1)*50,80,'t');
      | text(15,20,str);
  "Discrete On Delay  " : powerlib_extras/Discrete  Control Blocks/Discrete On//Off Delay  type_delay=On delay  delay=0.2  ic=0  Ts=dt
  Logical Operator2 : Logic  Inputs=3
  Logical Operator3 : Logic  Operator=NOT
  Logical Operator6 : Logic
  "Monostable: T2 " : powerlib_extras/Discrete  Control Blocks/Discrete Monostable  EdgeDetect=Rising  t_mono=T2  ic=0  Ts=dt
  "Off Delay " : powerlib_extras/Discrete  Control Blocks/Discrete On//Off Delay  type_delay=Off delay  delay=0.01  ic=0  Ts=dt
  On Delay: T1 : powerlib_extras/Discrete  Control Blocks/Discrete On//Off Delay  type_delay=On delay  delay=T1  ic=0  Ts=dt
  Ref1 (pu) : Relay  OnSwitchValue=-Ref1  OffSwitchValue=-(Ref1 + 0.1)
  minus : Gain  Gain=-1  SaturateOnIntegerOverflow=on  OutDataTypeStr=Inherit: Same as input  ParamDataTypeStr=Inherit: Same as input
  voltage sign (pole +) : Gain  Gain=sign  SaturateOnIntegerOverflow=on  OutDataTypeStr=Inherit: Same as input  ParamDataTypeStr=Inherit: Same as input
  Forced_alpha : Outport
  wires:
  "Monostable: T2 "/1 -> Forced_alpha/1
  On Delay: T1/1 -> "Monostable: T2 "/1
  Logical Operator2/1 -> On Delay: T1/1
  Logical Operator3/1 -> Logical Operator2/2
  Discrete Off Delay/1(OUT) -> Logical Operator3/1
  "Off Delay "/1 -> Logical Operator2/1
  Lock/1 -> Discrete Off Delay/1(IN)
  voltage sign (pole +)/1 -> minus/1
  VdL (pu)/1 -> voltage sign (pole +)/1  "VdL"
  Deblocked/1 -> "Discrete On Delay  "/1, Logical Operator2/3
  Ref1 (pu)/1 -> Data Type Conversion/1
  Logical Operator6/1 -> "Off Delay "/1
  "Discrete On Delay  "/1 -> Logical Operator6/2
  Data Type Conversion/1 -> Logical Operator6/1
  minus/1 -> Ref1 (pu)/1

== system Controls/Pole 1 Rectifier Control and Protection/Rectifier Protections/Low AC Voltage Detection (LACVD)/Enabled Subsystem ==
  note: Low AC Voltage Detection
  note: Silvano Casoria
      | Power System Laboratory, IREQ
      | Hydro-Quebec
  Uac (pu) : Inport
  Data Type Conversion2 : DataTypeConversion  OutDataTypeStr=double
  "Off Delay " : powerlib_extras/Discrete  Control Blocks/Discrete On//Off Delay  type_delay=Off delay  delay=0.009  ic=0  Ts=dt
  On Delay : powerlib_extras/Discrete  Control Blocks/Discrete On//Off Delay  type_delay=On delay  delay=0.014  ic=0  Ts=dt
  "On Delay " : powerlib_extras/Discrete  Control Blocks/Discrete On//Off Delay  type_delay=On delay  delay=0.001  ic=0  Ts=dt
  REF 1 (pu) : Constant  Value=Ref_1
  Relational Operator1 : RelationalOperator  Operator=<=
  Low_AC_Voltage : Outport
  wires:
  Data Type Conversion2/1 -> Low_AC_Voltage/1
  Uac (pu)/1 -> Relational Operator1/1
  On Delay/1 -> Data Type Conversion2/1
  REF 1 (pu)/1 -> Relational Operator1/2
  "Off Delay "/1 -> On Delay/1
  "On Delay "/1 -> "Off Delay "/1
  Relational Operator1/1 -> "On Delay "/1

== system Controls/Pole 2 Inverter Control and Protection/Inverter Current //Voltage//Gamma Controller /Current Regulator/Kp Linearisation ==
  note: Kp Linearization
  Alpha_lin : Inport
  Kp : Inport  Port=2
  Inv : Inport  Port=3
  Min_lin : Inport  Port=4
  Max_lin : Inport  Port=5
  Constant3 : Constant  Value=On_lin
  Data Type Conversion : DataTypeConversion  OutDataTypeStr=boolean
  Logical Operator : Logic  Operator=NOT
  Logical Operator1 : Logic  Operator=NOT
  Math Function : Math  Operator=reciprocal  SignedPower=on
  Prod2 : Product  Inputs=3  InputSameDT=on  SaturateOnIntegerOverflow=on  OutDataTypeStr=Inherit: Same as first input
  S6 : Subsystem  mask(Limiter with External Limits){}
      mask Display: disp('      Limiter\n')
  Switch : Switch  Threshold=0.5
  Switch1 : Switch  Threshold=0.5
  Trigonometric Function : Trigonometry
  Trigonometric Function1 : Trigonometry
  k : Gain  Gain=pi/180  SaturateOnIntegerOverflow=on  OutDataTypeStr=Inherit: Same as input  ParamDataTypeStr=Inherit: Same as input
  k1 : Gain  Gain=pi/180  SaturateOnIntegerOverflow=on  OutDataTypeStr=Inherit: Same as input  ParamDataTypeStr=Inherit: Same as input
  Kp_lin : Outport  InitialOutput=0
  wires:
  Data Type Conversion/1 -> Logical Operator1/1
  Constant3/1 -> Data Type Conversion/1
  Min_lin/1 -> S6/3(MIN), Switch/1
  Max_lin/1 -> S6/1(MAX), Switch/3
  Alpha_lin/1 -> S6/2(In)
  Math Function/1 -> Prod2/2
  Trigonometric Function1/1 -> Math Function/1
  k/1 -> Trigonometric Function1/1
  Kp/1 -> Prod2/3, Switch1/1
  Inv/1 -> Logical Operator/1
  Logical Operator/1 -> Switch/2
  Trigonometric Function/1 -> Prod2/1
  S6/1("  ") -> k/1
  k1/1 -> Trigonometric Function/1
  Switch/1 -> k1/1
  Switch1/1 -> Kp_lin/1
  Prod2/1 -> Switch1/3
  Logical Operator1/1 -> Switch1/2  "Off"

== system Controls/Pole 2 Inverter Control and Protection/Inverter Current //Voltage//Gamma Controller /Current Regulator/S16 ==
  note: INTEGRATOR with External limits & Reset & Hold
  note: Gain * dt
  Max : Inport
  Min : Inport  Port=2
  In : Inport  Port=3
  Reset : Inport  Port=4
  Hold : Inport  Port=5
  Reset Value : Inport  Port=6
  Gain1 : Gain  Gain=k*dt  SaturateOnIntegerOverflow=on  OutDataTypeStr=Inherit: Same as input  ParamDataTypeStr=Inherit: Same as input
  IC = ic : UnitDelay  InitialCondition=ic  SampleTime=dt  HasFrameUpgradeWarning=on
  Logical Operator4 : Logic  Operator=OR
  MinMax : MinMax  Inputs=2  InputSameDT=on  SaturateOnIntegerOverflow=on
  MinMax1 : MinMax  Function=max  Inputs=2  InputSameDT=on  SaturateOnIntegerOverflow=on
  S6 : Subsystem  mask(Limiter with External Limits){}
      mask Display: disp('      Limiter\n')
  Sum : Sum  InputSameDT=on  SaturateOnIntegerOverflow=on  OutDataTypeStr=Inherit: Same as first input
  Switch2 : Switch  Threshold=0.5
  Switch3 : Switch  Threshold=0.5
  Switch7 : Switch  Threshold=0.5
  Out : Outport  InitialOutput=0
  wires:
  Gain1/1 -> Sum/1
  In/1 -> Gain1/1
  Sum/1 -> S6/2(In)
  S6/1("  ") -> Out/1, IC = ic/1
  Hold/1 -> Logical Operator4/1
  Reset/1 -> Switch7/2, Logical Operator4/2
  Logical Operator4/1 -> Switch2/2, Switch3/2
  Switch2/1 -> MinMax/1
  Max/1 -> Switch2/3, MinMax/2
  Reset Value/1 -> Switch7/1
  MinMax/1 -> S6/1(MAX)
  MinMax1/1 -> S6/3(MIN)
  Switch3/1 -> MinMax1/1
  Min/1 -> Switch3/3, MinMax1/2
  IC = ic/1 -> Switch7/3
  Switch7/1 -> Switch2/1, Sum/2, Switch3/1

== system Controls/Pole 2 Inverter Control and Protection/Inverter Current //Voltage//Gamma Controller /Current Regulator/S6 ==
  note: Limiter
      | with external
      | limits
  MAX : Inport
  In : Inport  Port=2
  MIN : Inport  Port=3
  MinMax : MinMax  Function=max  Inputs=2  InputSameDT=on  SaturateOnIntegerOverflow=on
  MinMax1 : MinMax  Inputs=2  InputSameDT=on  SaturateOnIntegerOverflow=on
  "  " : Outport  InitialOutput=0
  wires:
  In/1 -> MinMax1/2
  MinMax/1 -> "  "/1
  MIN/1 -> MinMax/1
  MAX/1 -> MinMax1/1
  MinMax1/1 -> MinMax/2

== system Controls/Pole 2 Inverter Control and Protection/Inverter Current //Voltage//Gamma Controller /Gamma Error/S6 ==
  note: Limiter
      | with external
      | limits
  MAX : Inport
  In : Inport  Port=2
  MIN : Inport  Port=3
  MinMax : MinMax  Function=max  Inputs=2  InputSameDT=on  SaturateOnIntegerOverflow=on
  MinMax1 : MinMax  Inputs=2  InputSameDT=on  SaturateOnIntegerOverflow=on
  "  " : Outport  InitialOutput=0
  wires:
  MinMax1/1 -> MinMax/2
  MAX/1 -> MinMax1/1
  MIN/1 -> MinMax/1
  MinMax/1 -> "  "/1
  In/1 -> MinMax1/2

== system Controls/Pole 2 Inverter Control and Protection/Inverter Current //Voltage//Gamma Controller /Gamma Regulator/Gamma Regulator ==
  note: PI Regulator With external limits (Linearized Kp) (Discrete)
  Max_i : Inport
  Min_i : Inport  Port=2
  ERR : Inport  Port=3
  Max_pi : Inport  Port=4
  Min_pi : Inport  Port=5
  Alpha_lin : Inport  Port=6
  Max_lin : Inport  Port=7
  Min_lin : Inport  Port=8
  Inv : Inport  Port=9
  Kp : Inport  Port=10
  Ki : Inport  Port=11
  Ground : Ground
  KI (deg per pu per s) : Gain  Gain=Ki  SaturateOnIntegerOverflow=on  OutDataTypeStr=Inherit: Same as input  ParamDataTypeStr=Inherit: Same as input
  Kp (deg per pu) : Constant  Value=Kp
  Kp Linearisation : Subsystem
  Prod : Product  InputSameDT=on  SaturateOnIntegerOverflow=on  OutDataTypeStr=Inherit: Same as first input
  Prod1 : Product  InputSameDT=on  SaturateOnIntegerOverflow=on  OutDataTypeStr=Inherit: Same as first input
  S16 : Subsystem  mask(Integrator  With  External  Dynamic  Limits (Discrete)){k=1, ic=IC_i, st=pas}
      mask prompts: k "Gain:"; ic "Initial Condition:"; st "Sample time: (s)"
      mask Display: disp('Integrator\nwith\nExternal Limits\nGain & Reset & Hold\n(Discrete)')
  S6 : Subsystem  mask(Limiter with External Limits){}
      mask Display: disp('      Limiter\n')
  Sum : Sum  InputSameDT=on  SaturateOnIntegerOverflow=on  OutDataTypeStr=Inherit: Same as first input
  Alpha_ord : Outport  InitialOutput=0
  wires:
  Prod1/1 -> S16/3(In)
  Ki/1 -> Prod1/2
  Kp/1 -> Kp Linearisation/2(Kp)
  Alpha_lin/1 -> Kp Linearisation/1(Alpha_lin)
  S6/1("  ") -> Alpha_ord/1
  Kp Linearisation/1(Kp_lin) -> Prod/1
  Max_i/1 -> S16/1(Max)
  Min_i/1 -> S16/2(Min)
  Sum/1 -> S6/2(In)
  Max_pi/1 -> S6/1(MAX)
  Min_pi/1 -> S6/3(MIN)
  S16/1(Out) -> Sum/2
  ERR/1 -> Prod1/1, KI (deg per pu per s)/1, Prod/2
  Ground/1 -> S16/4(Reset), S16/5(Hold), S16/6(Reset Value)
  Inv/1 -> Kp Linearisation/3(Inv)
  Max_lin/1 -> Kp Linearisation/5(Max_lin)
  Min_lin/1 -> Kp Linearisation/4(Min_lin)
  Prod/1 -> Sum/1

== system Controls/Pole 2 Inverter Control and Protection/Inverter Current //Voltage//Gamma Controller /Voltage Dependant Current Order Limiter/PB_R ==
  note: Silvano Casoria
      | Laboratoire simulation de reseaux, IREQ
  note: LOW PASS Filter & RESET
      | (Zoh methode)
  "In " : Inport
  Reset : Inport  Port=2
  T : Inport  Port=3
  Constant : Constant  Value=dt
  IC= ic : UnitDelay  InitialCondition=ic  SampleTime=dt  HasFrameUpgradeWarning=on
  Math Function : Math  Operator=reciprocal  SignedPower=on
  Product : Product  Inputs=3  InputSameDT=on  SaturateOnIntegerOverflow=on  OutDataTypeStr=Inherit: Same as first input
  Sum : Sum  Inputs=+-  InputSameDT=on  SaturateOnIntegerOverflow=on  OutDataTypeStr=Inherit: Same as first input
  Sum1 : Sum  InputSameDT=on  SaturateOnIntegerOverflow=on
  Switch : Switch  Threshold=0.5
  Out : Outport  InitialOutput=0
  wires:
  IC= ic/1 -> Sum/2, Sum1/2
  "In "/1 -> Sum/1, Switch/1
  Reset/1 -> Switch/2
  Sum1/1 -> Out/1, Switch/3
  Switch/1 -> IC= ic/1
  Product/1 -> Sum1/1
  Sum/1 -> Product/2
  Math Function/1 -> Product/1
  T/1 -> Math Function/1
  Constant/1 -> Product/3

== system Controls/Pole 2 Inverter Control and Protection/Inverter Current //Voltage//Gamma Controller /Voltage Error/S6 ==
  note: Limiter
      | with external
      | limits
  MAX : Inport
  In : Inport  Port=2
  MIN : Inport  Port=3
  MinMax : MinMax  Function=max  Inputs=2  InputSameDT=on  SaturateOnIntegerOverflow=on
  MinMax1 : MinMax  Inputs=2  InputSameDT=on  SaturateOnIntegerOverflow=on
  "  " : Outport  InitialOutput=0
  wires:
  In/1 -> MinMax1/2
  MinMax/1 -> "  "/1
  MIN/1 -> MinMax/1
  MAX/1 -> MinMax1/1
  MinMax1/1 -> MinMax/2

== system Controls/Pole 2 Inverter Control and Protection/Inverter Current //Voltage//Gamma Controller /Voltage Regulator/Voltage Regulator ==
  note: PI Regulator With external limits (Linearized Kp) (Discrete)
  Max_i : Inport
  Min_i : Inport  Port=2
  ERR : Inport  Port=3
  Max_pi : Inport  Port=4
  Min_pi : Inport  Port=5
  Alpha_lin : Inport  Port=6
  Max_lin : Inport  Port=7
  Min_lin : Inport  Port=8
  Inv : Inport  Port=9
  Kp : Inport  Port=10
  Ki : Inport  Port=11
  Ground : Ground
  KI (deg per pu per s) : Gain  Gain=Ki  SaturateOnIntegerOverflow=on  OutDataTypeStr=Inherit: Same as input  ParamDataTypeStr=Inherit: Same as input
  Kp (deg per pu) : Constant  Value=Kp
  Kp Linearisation : Subsystem
  Prod : Product  InputSameDT=on  SaturateOnIntegerOverflow=on  OutDataTypeStr=Inherit: Same as first input
  Prod1 : Product  InputSameDT=on  SaturateOnIntegerOverflow=on  OutDataTypeStr=Inherit: Same as first input
  S16 : Subsystem  mask(Integrator  With  External  Dynamic  Limits (Discrete)){k=1, ic=IC_i, st=pas}
      mask prompts: k "Gain:"; ic "Initial Condition:"; st "Sample time: (s)"
      mask Display: disp('Integrator\nwith\nExternal Limits\nGain & Reset & Hold\n(Discrete)')
  S6 : Subsystem  mask(Limiter with External Limits){}
      mask Display: disp('      Limiter\n')
  Sum : Sum  InputSameDT=on  SaturateOnIntegerOverflow=on  OutDataTypeStr=Inherit: Same as first input
  Alpha_ord : Outport  InitialOutput=0
  wires:
  Prod1/1 -> S16/3(In)
  Ki/1 -> Prod1/2
  Kp/1 -> Kp Linearisation/2(Kp)
  Prod/1 -> Sum/1
  Min_lin/1 -> Kp Linearisation/4(Min_lin)
  Max_lin/1 -> Kp Linearisation/5(Max_lin)
  Inv/1 -> Kp Linearisation/3(Inv)
  Ground/1 -> S16/6(Reset Value), S16/5(Hold), S16/4(Reset)
  ERR/1 -> Prod1/1, Prod/2, KI (deg per pu per s)/1
  S16/1(Out) -> Sum/2
  Min_pi/1 -> S6/3(MIN)
  Max_pi/1 -> S6/1(MAX)
  Sum/1 -> S6/2(In)
  Min_i/1 -> S16/2(Min)
  Max_i/1 -> S16/1(Max)
  Kp Linearisation/1(Kp_lin) -> Prod/1
  S6/1("  ") -> Alpha_ord/1
  Alpha_lin/1 -> Kp Linearisation/1(Alpha_lin)

== system Controls/Pole 2 Inverter Control and Protection/Inverter Protections/Commutation Failure Prevention Control (CFPREV)/Enabled Subsystem ==
  note: Fast initialisation
      | for simulation
  note: Commutation failure Prevention Control (CFPREV)
  note: Silvano Casoria
      | Power System Laboratory, IREQ
      | Hydro-Quebec
  note: Ref. "A Novel Method to Mitigate Commutation Failures in HVDC Systems,"
      | Lidong Zhang, Lars Dofnas ABB Utilities Power System Technology,
      | Proceedings PowerCon 2002, Volume: 1 , 13-17 Oct. 2002,  Page(s): 51-56 vol.1
  Uabc (pu) : Inport
  Enable : EnablePort
  AB_LEVEL : Constant  Value=ab_level
  ALPFA_BETA_SUM : Fcn  Expr=sqrt(u[1]^2+u[2]^2)
  ALPFA_BETA_SUM1 : Fcn  Expr=abs(u[3]) * 3
  C : Constant  Value=filt_tc
  C1 : Constant  Value=1/(fn)
  CLARK : Subsystem
  Gain : Gain  Gain=ab_gain  SaturateOnIntegerOverflow=on  OutDataTypeStr=Inherit: Same as input  ParamDataTypeStr=Inherit: Same as input
  "Gain  " : Gain  Gain=z_gain  SaturateOnIntegerOverflow=on  OutDataTypeStr=Inherit: Same as input  ParamDataTypeStr=Inherit: Same as input
  Ground : Ground
  LP T= 0.03 : powerlib_extras/Discrete  Control Blocks/Discrete 1st-Order Filter  FilterType=Lowpass  Tc=0.03  Ts=Ts  Initialize=off  Vac_Init=[0.8 -25 60]*0  Vdc_Init=filt_ic  PlotResponse=off  param1=[1 500 0.1]
  Max: 1 pu Min = 0 : Saturate  UpperLimit=1.0  LowerLimit=0
  MinMax2 : MinMax  Function=max  InputSameDT=on  SaturateOnIntegerOverflow=on
  MinMax3 : MinMax  Function=max  Inputs=2  InputSameDT=on  SaturateOnIntegerOverflow=on
  MinMax4 : MinMax  Function=max  Inputs=2  InputSameDT=on  SaturateOnIntegerOverflow=on
  MinMax5 : MinMax  Function=max  InputSameDT=on  SaturateOnIntegerOverflow=on
  PB_R : Subsystem  mask(Low Pass Filter With Reset (discrete: Zoh method, Forward Euler)){ic=1, dt=Ts}
      mask prompts: ic "Initial condition:"; dt "Sample time (s)"
      mask help:
      | The output will be reset to the input value (Time constant = 0)  during the input (2) is True. The Time constant (T) is defined by
      | input (3).
      mask Display:
      | plot(0,0,100,100,[90,80,70,60,50,40,29,20,10],[60,55,52,55,60,65,67,65,60],[89,80,71,60,50,40,30,20,10],[40,35,32,35,40,45,47,45,40],[56,44],[70,50]);
      | disp('\n\nD')
  Relational Operator : RelationalOperator  Operator=>  InputSameDT=off
  Relational Operator1 : RelationalOperator  Operator=>  InputSameDT=off
  Sum : Sum  Inputs=+-  SaturateOnIntegerOverflow=on
  Switch : Switch  Threshold=0.5  InputSameDT=off
  Switch1 : Switch  Threshold=0.5  InputSameDT=off
  Switch2 : Switch  Threshold=0.5  InputSameDT=off
  T_ss : Step  Time=T_ss  Before=1  After=0  SampleTime=Ts
  Tapped Delay : simulink/Discrete/Tapped Delay  vinit=0.0  samptime=Ts  NumDelays=fix(T_periode/Ts)  DelayOrder=Newest  includeCurrent=off
  Tapped Delay1 : simulink/Discrete/Tapped Delay  vinit=0.0  samptime=Ts  NumDelays=fix(T_periode/Ts)  DelayOrder=Newest  includeCurrent=off
  ZERO : Constant  Value=0
  ZERO1 : Constant  Value=0
  Z_LEVEL : Constant  Value=z_level
  AMIN_CFPREV (deg) : Outport
  wires:
  Tapped Delay/1 -> MinMax5/1
  Ground/1 -> PB_R/2(Reset)
  C1/1 -> Switch2/1
  T_ss/1 -> Switch2/2
  C/1 -> Switch2/3
  Switch2/1 -> PB_R/3(T)
  PB_R/1(Out) -> Sum/1
  Uabc (pu)/1 -> CLARK/1(abc)
  CLARK/1(ab0) -> ALPFA_BETA_SUM1/1, ALPFA_BETA_SUM/1
  Switch1/1 -> MinMax3/2  "Z MIN"
  Switch/1 -> MinMax3/1  "AB MIN"
  ZERO1/1 -> Switch1/3
  "Gain  "/1 -> Switch1/1  "Z_AMIN"
  Relational Operator1/1 -> Switch1/2  "Z_DET"
  Max: 1 pu Min = 0/1 -> "Gain  "/1
  MinMax2/1 -> Max: 1 pu Min = 0/1
  Tapped Delay1/1 -> MinMax2/1
  Z_LEVEL/1 -> Relational Operator1/2
  ALPFA_BETA_SUM1/1 -> Tapped Delay1/1, Relational Operator1/1  "Z_DIFF"
  ZERO/1 -> Switch/3
  Gain/1 -> Switch/1  "AB_AMIN"
  MinMax5/1 -> Gain/1
  Relational Operator/1 -> Switch/2  "AB_DET"
  AB_LEVEL/1 -> Relational Operator/2
  Sum/1 -> Tapped Delay/1, Relational Operator/1
  ALPFA_BETA_SUM/1 -> PB_R/1("In "), Sum/2
  MinMax3/1 -> MinMax4/2, LP T= 0.03/1
  LP T= 0.03/1 -> MinMax4/1
  MinMax4/1 -> AMIN_CFPREV (deg)/1

== system Controls/Pole 2 Inverter Control and Protection/Inverter Protections/Low AC Voltage Detection (LACVD)/Enabled Subsystem ==
  note: Low AC Voltage Detection
  note: Silvano Casoria
      | Power System Laboratory, IREQ
      | Hydro-Quebec
  Uac (pu) : Inport
  "Off Delay " : powerlib_extras/Discrete  Control Blocks/Discrete On//Off Delay  type_delay=Off delay  delay=0.009  ic=0  Ts=dt
  On Delay : powerlib_extras/Discrete  Control Blocks/Discrete On//Off Delay  type_delay=On delay  delay=0.014  ic=0  Ts=dt
  "On Delay " : powerlib_extras/Discrete  Control Blocks/Discrete On//Off Delay  type_delay=On delay  delay=0.001  ic=0  Ts=dt
  REF 1 (pu) : Constant  Value=Ref_1
  Relational Operator1 : RelationalOperator  Operator=<=
  Low_AC_Voltage : Outport
  wires:
  Uac (pu)/1 -> Relational Operator1/1
  On Delay/1 -> Low_AC_Voltage/1
  REF 1 (pu)/1 -> Relational Operator1/2
  "Off Delay "/1 -> On Delay/1
  "On Delay "/1 -> "Off Delay "/1
  Relational Operator1/1 -> "On Delay "/1

== system Controls/Pole 2 Rectifier Control and Protection/Rectifier Controller/Current Regulator/Kp Linearisation ==
  note: Kp Linearization
  Alpha_lin : Inport
  Kp : Inport  Port=2
  Inv : Inport  Port=3
  Min_lin : Inport  Port=4
  Max_lin : Inport  Port=5
  Constant3 : Constant  Value=On_lin
  Data Type Conversion : DataTypeConversion  OutDataTypeStr=boolean
  Logical Operator : Logic  Operator=NOT
  Logical Operator1 : Logic  Operator=NOT
  Math Function : Math  Operator=reciprocal  SignedPower=on
  Prod2 : Product  Inputs=3  InputSameDT=on  SaturateOnIntegerOverflow=on  OutDataTypeStr=Inherit: Same as first input
  S6 : Subsystem  mask(Limiter with External Limits){}
      mask Display: disp('      Limiter\n')
  Switch : Switch  Threshold=0.5
  Switch1 : Switch  Threshold=0.5
  Trigonometric Function : Trigonometry
  Trigonometric Function1 : Trigonometry
  k : Gain  Gain=pi/180  SaturateOnIntegerOverflow=on  OutDataTypeStr=Inherit: Same as input  ParamDataTypeStr=Inherit: Same as input
  k1 : Gain  Gain=pi/180  SaturateOnIntegerOverflow=on  OutDataTypeStr=Inherit: Same as input  ParamDataTypeStr=Inherit: Same as input
  Kp_lin : Outport  InitialOutput=0
  wires:
  Data Type Conversion/1 -> Logical Operator1/1
  Constant3/1 -> Data Type Conversion/1
  Min_lin/1 -> S6/3(MIN), Switch/1
  Max_lin/1 -> S6/1(MAX), Switch/3
  Alpha_lin/1 -> S6/2(In)
  Math Function/1 -> Prod2/2
  Trigonometric Function1/1 -> Math Function/1
  k/1 -> Trigonometric Function1/1
  Kp/1 -> Prod2/3, Switch1/1
  Inv/1 -> Logical Operator/1
  Logical Operator/1 -> Switch/2
  Trigonometric Function/1 -> Prod2/1
  S6/1("  ") -> k/1
  k1/1 -> Trigonometric Function/1
  Switch/1 -> k1/1
  Switch1/1 -> Kp_lin/1
  Prod2/1 -> Switch1/3
  Logical Operator1/1 -> Switch1/2  "Off"
